simulink model "simulacao_sem_linearizar"  (R2017a)
settings: Solver=VariableStepAuto  StartTime=0.0  StopTime=10.0  RelTol=1e-3
values from neighbouring files (symbols this model uses):
  a = -9128    [prepare_y_prbs.m]
undefined symbols (not defined in the file or in its folder): g, m
settings Model: Creator=Mateus  LastModifiedBy=Mateus

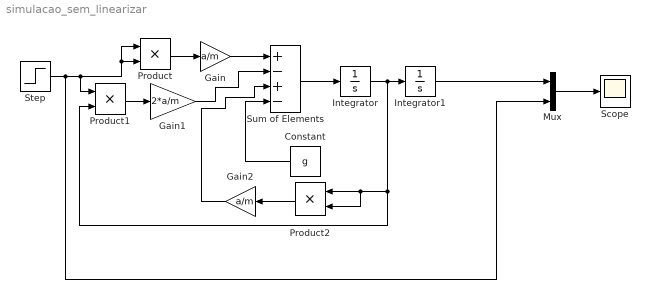
== system simulacao_sem_linearizar ==
  Constant : Constant  Value=g
  Gain : Gain  Gain=a/m
  Gain1 : Gain  Gain=2*a/m
  Gain2 : Gain  Gain=a/m
  Integrator : Integrator
  Integrator1 : Integrator
  Mux : Mux  Inputs=2
  Product : Product
  Product1 : Product
  Product2 : Product
  Scope : Scope
  Step : Step  Time=0  After=15  SampleTime=0
  Sum of Elements : Sum  Inputs=+-+-
  wires:
  Mux/1 -> Scope/1
  Step/1 -> Mux/2, Product1/1, Product/1, Product/2
  Product/1 -> Gain/1
  Integrator/1 -> Product2/2, Product2/1, Product1/2, Integrator1/1
  Sum of Elements/1 -> Integrator/1
  Gain/1 -> Sum of Elements/1
  Product1/1 -> Gain1/1
  Gain1/1 -> Sum of Elements/2
  Product2/1 -> Gain2/1
  Gain2/1 -> Sum of Elements/3
  Constant/1 -> Sum of Elements/4
  Integrator1/1 -> Mux/1
